simulink model "p4"  (R2020a)
settings: Solver=VariableStepAuto  StartTime=0.0  StopTime=10.0  RelTol=1e-3
model workspace (MAT data in the model file):
  A = Simulink.Parameter
  A.Value = 0.4
  A.DataType = 'auto'
  A.Dimensions = [1 1]
  B = Simulink.Parameter
  B.Value = 0.5
  B.DataType = 'auto'
  B.Dimensions = [1 1]
  C = Simulink.Parameter
  C.Value = -0.25
  C.DataType = 'auto'
  C.Dimensions = [1 1]
settings Model: Creator=007  LastModifiedBy=007

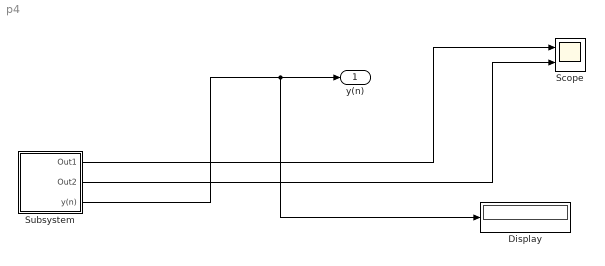
== system p4 ==
  Display : Display
  Scope : Scope  NumInputPorts=2
  Subsystem : Subsystem
  y(n) : Outport
  wires:
  Subsystem/1(Out1) -> Scope/1
  Subsystem/3(y(n)) -> Display/1, y(n)/1
  Subsystem/2(Out2) -> Scope/2

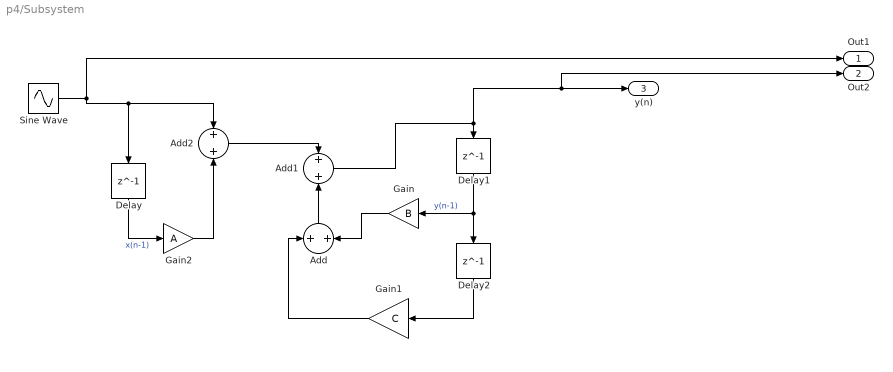
== system p4/Subsystem ==
  Add : Sum
  Add1 : Sum
  Add2 : Sum
  Delay : Delay  DelayLength=1
  Delay1 : Delay  DelayLength=1
  Delay2 : Delay  DelayLength=1
  Gain : Gain  Gain=B
  Gain1 : Gain  Gain=C
  Gain2 : Gain  Gain=A
  Sine Wave : Sin  SampleTime=0
  Out1 : Outport
  Out2 : Outport  Port=2
  y(n) : Outport  Port=3
  wires:
  Add1/1 -> y(n)/1, Out2/1, Delay1/1
  Gain/1 -> Add/2
  Add/1 -> Add1/2
  Delay/1 -> Gain2/1  "x(n-1)"
  Gain1/1 -> Add/1
  Add2/1 -> Add1/1
  Sine Wave/1 -> Add2/1, Delay/1, Out1/1
  Delay1/1 -> Delay2/1, Gain/1  "y(n-1)"
  Delay2/1 -> Gain1/1
  Gain2/1 -> Add2/2
